simulink model "cruise_control_model1"  (R2018a)
settings: Solver=ode45  StartTime=0.0  StopTime=120  RelTol=1e-3
settings Model: Creator=sansh  LastModifiedBy=3
settings CodeAppCC: StateflowObjectComments=on

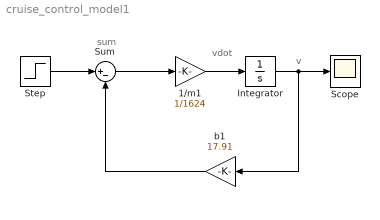
== system cruise_control_model1 ==
  note: v
  note: vdot
  note: sum
  1/m1 : Gain  Gain=1/1624
  Integrator : Integrator
  Scope : Scope
  Step : Step  Time=0  After=26.8  SampleTime=0
  Sum : Sum  Inputs=|+-
  b1 : Gain  Gain=17.91
  wires:
  Integrator/1 -> Scope/1, b1/1
  Sum/1 -> 1/m1/1
  b1/1 -> Sum/2
  Step/1 -> Sum/1
  1/m1/1 -> Integrator/1
